simulink subsystem "cart_pole_system_dynamics"  (R2023a)
settings: Solver=VariableStepAuto  StartTime=0.0  StopTime=10.0  RelTol=1e-3
values from neighbouring files (symbols this model uses):
  g = 9.80665    [Init_Multi.m]
settings Model: Creator=divij  LastModifiedBy=divij

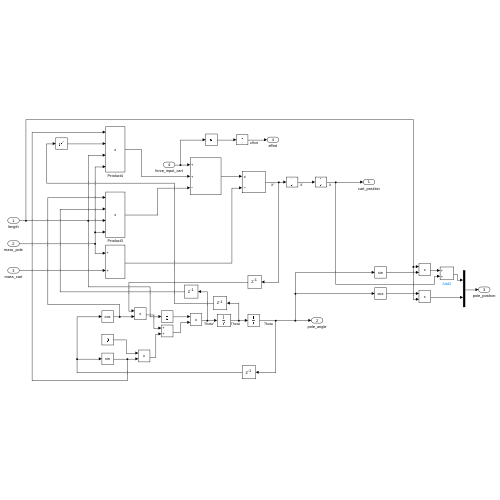
[thumbnail: Simulink's stored preview of the top-level diagram]
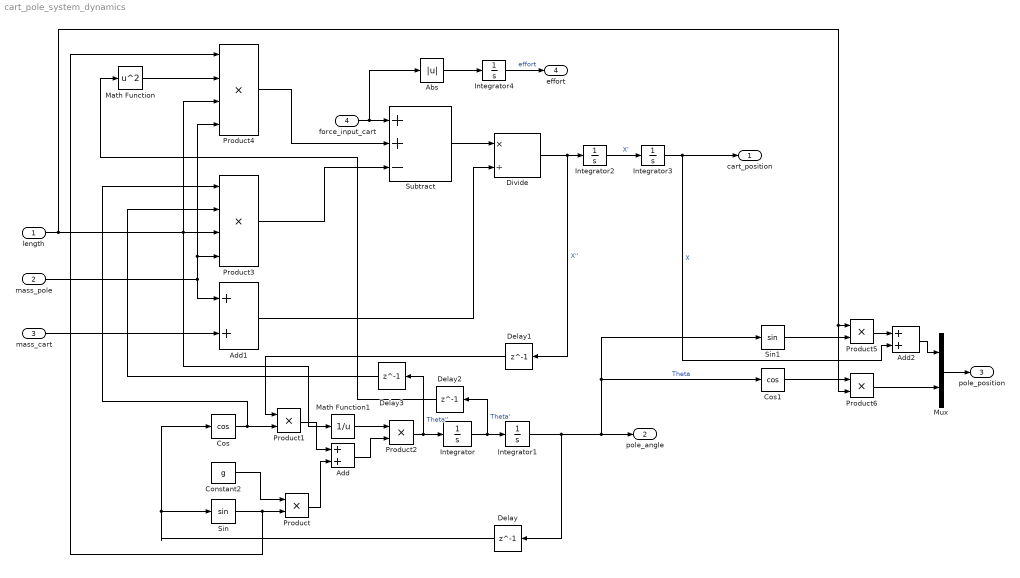
== system cart_pole_system_dynamics ==
  length : Inport
  mass_pole : Inport  Port=2
  mass_cart : Inport  Port=3
  force_input_cart : Inport  Port=4
  Abs : Abs  SaturateOnIntegerOverflow=off
  Add : Sum
  Add1 : Sum
  Add2 : Sum
  Constant2 : Constant  Value=g
  Cos : Trigonometry  Operator=cos
  Cos1 : Trigonometry  Operator=cos
  Delay{,1..3} (4 alike) : Delay  DelayLength=1  InitialCondition=0
  Divide : Product  Inputs=*/
  Integrator{,1..2,4} (4 alike) : Integrator
  Integrator3 : Integrator  UpperSaturationLimit=10  LowerSaturationLimit=-10
  Math Function : Math  Operator=square
  Math Function1 : Math  Operator=reciprocal
  Mux : Mux  Inputs=2
  Product{,1..2,5..6} (5 alike) : Product
  Product3 : Product  Inputs=4
  Product4 : Product  Inputs=4
  Sin : Trigonometry
  Sin1 : Trigonometry
  Subtract : Sum  Inputs=++-
  cart_position : Outport
  pole_angle : Outport  Port=2
  pole_position : Outport  Port=3
  effort : Outport  Port=4
  wires:
  Add1/1 -> Divide/2
  force_input_cart/1 -> Abs/1, Subtract/1
  Product2/1 -> Integrator/1, Delay3/1  "Theta''"
  mass_pole/1 -> Product3/4, Product4/4, Add1/1
  mass_cart/1 -> Add1/2
  Subtract/1 -> Divide/1
  Math Function1/1 -> Product2/1
  Product3/1 -> Subtract/3
  Constant2/1 -> Product/1
  Cos/1 -> Product1/2, Product3/1
  Integrator/1 -> Integrator1/1, Delay2/1  "Theta'"
  Product1/1 -> Add/1
  Product/1 -> Add/2
  Integrator3/1 -> cart_position/1, Add2/2  "X"
  length/1 -> Product3/3, Product4/3, Math Function1/1, Product6/2, Product5/1
  Integrator1/1 -> Cos1/1, Sin1/1, pole_angle/1, Delay/1  "Theta"
  Divide/1 -> Integrator2/1, Delay1/1  "X''"
  Integrator2/1 -> Integrator3/1  "X'"
  Sin/1 -> Product/2, Product4/1
  Math Function/1 -> Product4/2
  Add/1 -> Product2/2
  Product4/1 -> Subtract/2
  Delay/1 -> Cos/1, Sin/1
  Delay1/1 -> Product1/1
  Delay2/1 -> Math Function/1
  Delay3/1 -> Product3/2
  Sin1/1 -> Product5/2
  Cos1/1 -> Product6/1
  Product6/1 -> Mux/2
  Product5/1 -> Add2/1
  Add2/1 -> Mux/1
  Mux/1 -> pole_position/1
  Integrator4/1 -> effort/1  "effort"
  Abs/1 -> Integrator4/1
